simulink model "SEM_model"  (R2021a)
settings: Solver=VariableStepAuto  StartTime=0.0  StopTime=10.0  RelTol=1e-3
values from neighbouring files (symbols this model uses):
  alpha_1 = C_fr/r_ds - C_mfs/r_mfs    (= 2.23088597989e-13)    [CalcEquilibrium.m]    (also in linearizeMatrix.m = sym('alpha_1', 'real'))
  alpha_2 = C_mfs/r_ds - C_ds/r_mfs    (= -1.0557010055e-12)    [CalcEquilibrium.m]    (also in linearizeMatrix.m = sym('alpha_2', 'real'))
  alpha_3 = C_mfs/r_fr - C_fr/r_mfs    (= -4.94682230869e-13)    [CalcEquilibrium.m]    (also in linearizeMatrix.m = sym('alpha_3', 'real'))
  alpha_4 = C_ds/r_fr - C_mfs/r_mfs    (= -1.62034463591e-13)    [CalcEquilibrium.m]    (also in linearizeMatrix.m = sym('alpha_4', 'real'))
  beta = 10    [CalcEquilibrium.m]    (also in linearizeMatrix.m = sym('beta', 'real'))
  C_fr = C_lfr + C_mfs    (= 2.1e-07)    [CalcEquilibrium.m]    (also in linearizeMatrix.m = sym('C_fr', {'positive', 'real'}))
  C_mfs = 82e-9    (= 8.2e-08)    [CalcEquilibrium.m]    (also in linearizeMatrix.m = sym('C_mfs', {'positive', 'real'}))
  C_qs = 512e-9    (= 5.12e-07)    [CalcEquilibrium.m]    (also in linearizeMatrix.m = sym('C_qs', {'positive', 'real'}))
  gamma = 1 / (C_ds * C_fr - C_mfs^2)    (= 9.92102861225e+12)    [CalcEquilibrium.m]    (also in linearizeMatrix.m = sym('gamma', 'real'))
  I_fr = Q_ds*gamma*alpha_3+Q_fr*gamma*alpha_4    (= 0.0113488975357)    [CalcEquilibrium.m]    (also in linearizeMatrix.m = sym('I_fr', {'real'}))
  J = 3.1e6    (= 3100000)    [CalcEquilibrium.m]    (also in linearizeMatrix.m = sym('J', {'positive', 'real'}))
  L_dc = 12    [CalcEquilibrium.m]    (also in linearizeMatrix.m = sym('L_dc', {'positive', 'real'}))
  M_d = sym('M_d', {'real'})    [linearizeMatrix.m]
  M_fe = sym('M_fe', {'real'})    [linearizeMatrix.m]
  M_q = sym('M_q', {'real'})    [linearizeMatrix.m]
  N = double(table2array(params(17,2)))    [CalcBaseVals.m]    (also in CalcEquilibrium.m = 10; linearizeMatrix.m = sym('N', {'positive', 'real', 'integer'}))
  r_dc = 12    [CalcEquilibrium.m]    (also in linearizeMatrix.m = sym('r_dc', {'positive', 'real'}))
  tau_1 = r_qs * C_qs    (= 0.257024)    [CalcEquilibrium.m]    (also in linearizeMatrix.m = sym('tau_1', 'real'))
  Tor_l = sym('Tor_l', {'real'})    [linearizeMatrix.m]
  V_in = double(table2array(params(7,2)))    [CalcBaseVals.m]    (also in linearizeMatrix.m = sym('V_in', {'real'}))
  z = double(table2array(params(12,2)))    [CalcBaseVals.m]    (also in CalcEquilibrium.m = 96; linearizeMatrix.m = sym('z', {'positive', 'real', 'integer'}))
undefined symbols (not defined in the file or in its folder): DiscIntNeverNeededParam
settings Model: Creator=divad  LastModifiedBy=divad

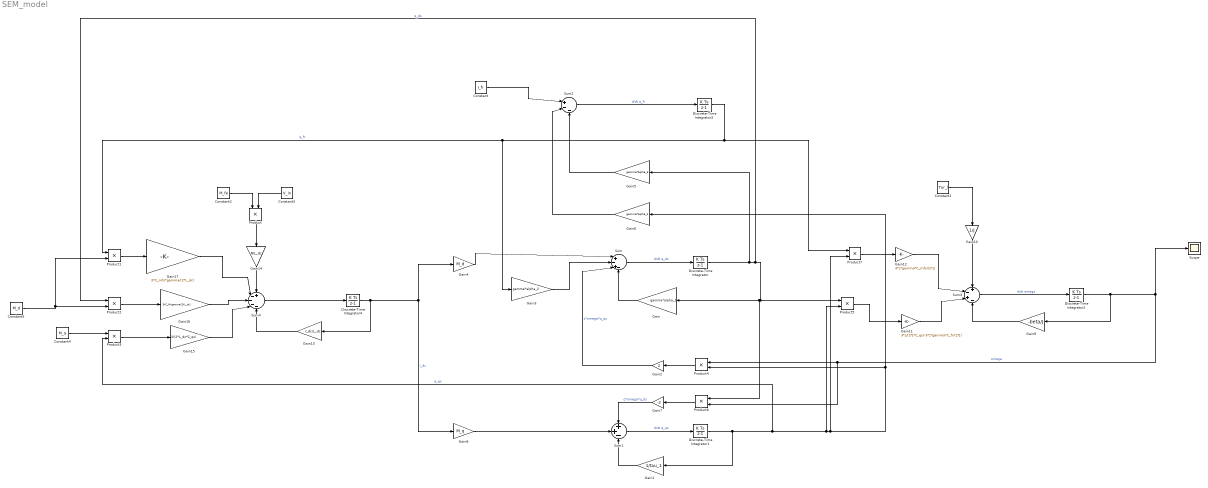
== system SEM_model ==
  Constant : Constant  Value=I_fr
  Constant1 : Constant  Value=Tor_l
  Constant2 : Constant  Value=M_fe
  Constant3 : Constant  Value=V_in
  Constant4 : Constant  Value=M_q
  Constant5 : Constant  Value=M_d
  Discrete-Time Integrator{,1..4} (5 alike) : DiscreteIntegrator  SampleTime=-1  ICPrevOutput=DiscIntNeverNeededParam  ICPrevScaledInput=DiscIntNeverNeededParam
  Gain : Gain  Gain=gamma*alpha_1
  Gain1 : Gain  Gain=1/tau_1
  Gain10 : Gain  Gain=1/J
  Gain11 : Gain  Gain=3*z/(2*J*C_qs)-3*z*gamma*C_fr/(2*J)
  Gain12 : Gain  Gain=3*z*gamma*C_mfs/(2*J)
  Gain13 : Gain  Gain=r_dc/L_dc
  Gain14 : Gain  Gain=N/L_dc
  Gain15 : Gain  Gain=3/(2*L_dc*C_qs)
  Gain16 : Gain  Gain=3*C_fr*gamma/(2*L_dc)
  Gain17 : Gain  Gain=3*C_mfs*gamma/(2*L_dc)
  Gain2 : Gain  Gain=z
  Gain3 : Gain  Gain=gamma*alpha_2
  Gain4 : Gain  Gain=M_d
  Gain5 : Gain  Gain=gamma*alpha_3
  Gain6 : Gain  Gain=gamma*alpha_4
  Gain7 : Gain  Gain=-z
  Gain8 : Gain  Gain=M_q
  Gain9 : Gain  Gain=-beta/J
  Product{,1..7} (8 alike) : Product
  Scope : Scope
  Sum : Sum  Inputs=|+-+-
  Sum1 : Sum  Inputs=++-
  Sum2 : Sum  Inputs=|+--
  Sum3 : Sum  Inputs=+-+-
  Sum4 : Sum  Inputs=+----
  wires:
  Sum/1 -> Discrete-Time Integrator/1  "d/dt q_ds"
  Discrete-Time Integrator/1 -> Gain5/1, Product2/1, Product5/1, Product6/1, Gain/1  "q_ds"
  Gain/1 -> Sum/4
  Sum1/1 -> Discrete-Time Integrator1/1  "d/dt q_qs"
  Discrete-Time Integrator1/1 -> Product3/2, Product7/2, Product4/2, Gain6/1, Product5/2, Gain1/1  "q_qs"
  Gain1/1 -> Sum1/3
  Gain2/1 -> Sum/3  "z*omega*q_qs"
  Sum2/1 -> Discrete-Time Integrator3/1  "d/dt q_fr"
  Gain3/1 -> Sum/2
  Sum3/1 -> Discrete-Time Integrator2/1  "d/dt omega"
  Product4/1 -> Gain2/1
  Discrete-Time Integrator2/1 -> Gain9/1, Scope/1, Product6/2, Product4/1  "omega"
  Discrete-Time Integrator3/1 -> Product7/1, Product1/1, Gain3/1  "q_fr"
  Sum4/1 -> Discrete-Time Integrator4/1
  Gain4/1 -> Sum/1
  Discrete-Time Integrator4/1 -> Gain13/1, Gain8/1, Gain4/1  "i_dc"
  Constant/1 -> Sum2/1
  Gain5/1 -> Sum2/3
  Gain6/1 -> Sum2/2
  Gain8/1 -> Sum1/2
  Product6/1 -> Gain7/1
  Gain7/1 -> Sum1/1  "-z*omega*q_ds"
  Gain9/1 -> Sum3/4
  Gain10/1 -> Sum3/1
  Constant1/1 -> Gain10/1
  Product5/1 -> Gain11/1
  Gain11/1 -> Sum3/3
  Gain12/1 -> Sum3/2
  Product7/1 -> Gain12/1
  Gain13/1 -> Sum4/5
  Gain14/1 -> Sum4/1
  Product3/1 -> Gain15/1
  Constant4/1 -> Product3/1
  Gain15/1 -> Sum4/4
  Gain16/1 -> Sum4/3
  Product2/1 -> Gain16/1
  Constant5/1 -> Product2/2, Product1/2
  Gain17/1 -> Sum4/2
  Product1/1 -> Gain17/1
  Product/1 -> Gain14/1
  Constant3/1 -> Product/2
  Constant2/1 -> Product/1
